simulink model "Sum2"  (R2017b)
settings: Solver=FixedStepDiscrete  StartTime=0.0  StopTime=10.0  FixedStep=0.200000  RelTol=1e-3
settings Model: Creator=hbourbou  LastModifiedBy=hbourbou
settings DataIOCC: SaveFormat=StructureWithTime
settings OptimizationCC: LifeSpan=inf
settings DebuggingCC: SFExecutionAtInitializationDiag=none
settings HardwareCC: ProdBitPerSizeT=32  ProdBitPerPtrDiffT=32  ProdWordSize=32  ProdHWDeviceType=Specified
settings CodeAppCC: StateflowObjectComments=on

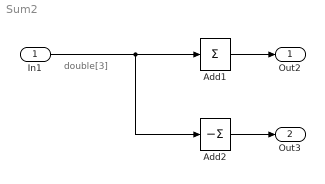
== system Sum2 ==
  note: double[3]
  In1 : Inport  OutDataTypeStr=double  PortDimensions=3
  Add1 : Sum  Inputs=+
  Add2 : Sum  Inputs=-
  Out2 : Outport
  Out3 : Outport  Port=2
  wires:
  Add1/1 -> Out2/1
  In1/1 -> Add2/1, Add1/1
  Add2/1 -> Out3/1
